simulink model "Prueba_Control_Cuadrupedo_Fisico_Imanes"  (R2025b)
settings: Solver=FixedStepAuto  StartTime=0.0  StopTime=inf  FixedStep=0.01  RelTol=1e-3
values from neighbouring files (symbols this model uses):
  f = figure('Color','w',            'Position',[300 300 900 220],            'Name','Joint Velocity Statistics')    [TABLE.m]
undefined symbols (not defined in the file or in its folder): DiscIntNeverNeededParam
libraries: instrumentlib x2, svdutilitieslib x1, simulink_extras x1
settings Model: PacingRate=0.300000  Creator=ketze  LastModifiedBy=ketze

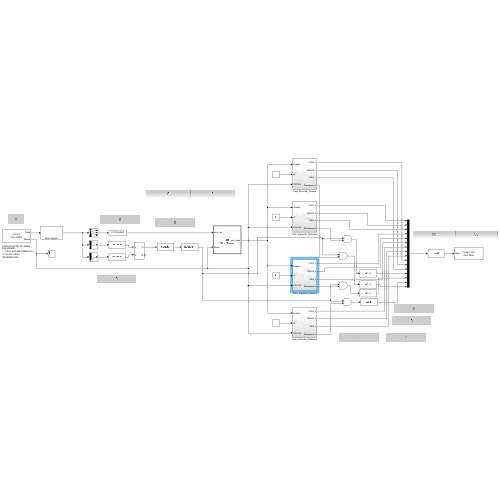
[thumbnail: Simulink's stored preview of the top-level diagram]
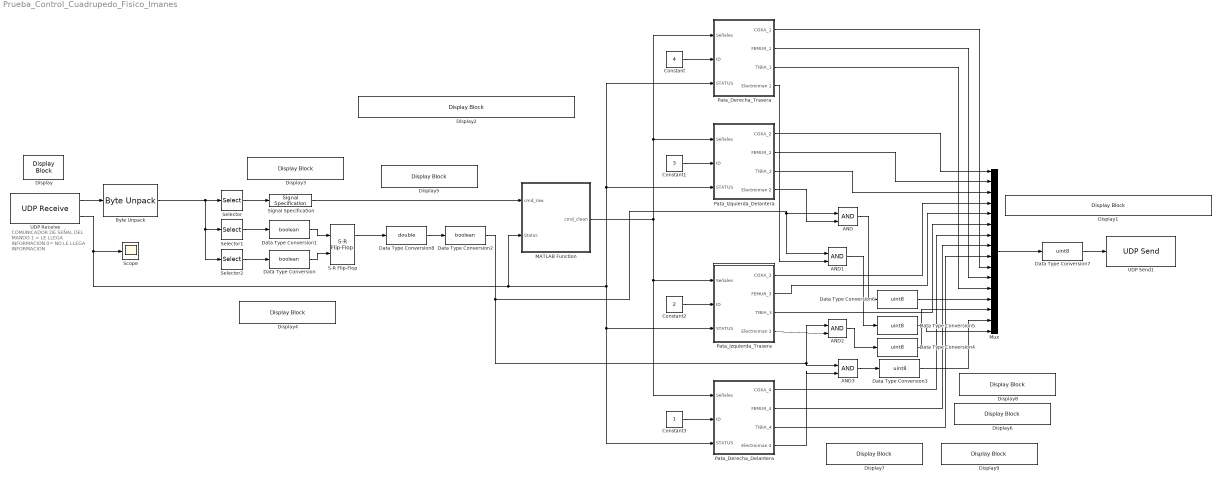
== system Prueba_Control_Cuadrupedo_Fisico_Imanes ==
  note: COMUNICADOR DE SEÑAL DEL MANDO
      | 1 = LE LLEGA INFORMACION
      | 0= NO LE LLEGA INFORMACION
  AND{,1..3} (4 alike) : Logic  IconShape=distinctive  AllPortsSameDT=off  OutDataTypeStr=boolean
  Byte Unpack : svdutilitieslib/Byte Unpack  dimensions={[5]}  datatypes={'double'}  byteAlign=1  blockPlatform=arduinoert
  Constant : Constant  Value=4
  Constant1 : Constant  Value=3
  Constant2 : Constant  Value=2
  Constant3 : Constant
  Data Type Conversion : DataTypeConversion  OutDataTypeStr=boolean  SaturateOnIntegerOverflow=off  RndMeth=Floor
  Data Type Conversion1 : DataTypeConversion  OutDataTypeStr=boolean  SaturateOnIntegerOverflow=off  RndMeth=Floor
  Data Type Conversion2 : DataTypeConversion  OutDataTypeStr=boolean  SaturateOnIntegerOverflow=off  RndMeth=Floor
  Data Type Conversion{3..7} (5 alike) : DataTypeConversion  OutDataTypeStr=uint8  SaturateOnIntegerOverflow=off  RndMeth=Floor
  Data Type Conversion8 : DataTypeConversion  OutDataTypeStr=double  SaturateOnIntegerOverflow=off  RndMeth=Floor
  Display{,1..9} (10 alike) : DisplayBlock  LabelPosition=Hide  Transparency=1  GridColor=[0.502, 0.502, 0.502]
  MATLAB Function : MATLAB Function  TreatAsAtomicUnit=on
  Mux : Mux  Inputs=16
  Pata_Derecha_Delantera : Subsystem
  Pata_Derecha_Trasera : Subsystem
  Pata_Izquierda_Delantera : Subsystem
  Pata_Izquierda_Trasera : Subsystem
  S-R Flip-Flop : simulink_extras/Flip Flops/S-R Flip-Flop  initial_condition=0
  Scope : Scope
  Selector : Selector  InputPortWidth=5  IndexOptions=Index vector (dialog)  Indices=[1 2 3]  OutputSizes=1
  Selector1 : Selector  InputPortWidth=5  IndexOptions=Index vector (dialog)  Indices=[4]  OutputSizes=1
  Selector2 : Selector  InputPortWidth=5  IndexOptions=Index vector (dialog)  Indices=[5]  OutputSizes=1
  Signal Specification : SignalSpecification  Dimensions=3
  UDP Receive : instrumentlib/UDP Receive  LocalAddress=0.0.0.0  LocalPort=25000  EnablePortSharing=off  Host=0.0.0.0  Port=9090  GetLatestData=off  DataSize=40  DataType=uint8  ASCIIFormatting=%f,  Terminator=LF  CustomTerminator=10  ByteOrder=big-endian  EnableBlockingMode=off  Timeout=10  SampleTime=0.02  SimulateUsing=Interpreted execution
  UDP Send1 : instrumentlib/UDP Send  Host=10.46.7.104  Port=5000  LocalAddress=0.0.0.0  LocalPort=-1  EnablePortSharing=off  OutputDatagramPacketSize=512  ByteOrder=big-endian  EnableBlockingMode=on  SimulateUsing=Interpreted execution
  wires:
  Mux/1 -> Data Type Conversion7/1
  Signal Specification/1 -> MATLAB Function/1(cmd_raw)
  UDP Receive/2 -> Scope/1, Pata_Derecha_Trasera/3(STATUS), Pata_Izquierda_Delantera/3(STATUS), Pata_Derecha_Delantera/3(STATUS), Pata_Izquierda_Trasera/3(STATUS), MATLAB Function/2(Status)
  UDP Receive/1 -> Byte Unpack/1
  Constant/1 -> Pata_Derecha_Trasera/2(ID)
  Constant1/1 -> Pata_Izquierda_Delantera/2(ID)
  Constant2/1 -> Pata_Izquierda_Trasera/2(ID)
  Constant3/1 -> Pata_Derecha_Delantera/2(ID)
  MATLAB Function/1(cmd_clean) -> Pata_Derecha_Trasera/1(Señales), Pata_Izquierda_Delantera/1(Señales), Pata_Derecha_Delantera/1(Señales), Pata_Izquierda_Trasera/1(Señales)
  Pata_Izquierda_Delantera/1(COXA_2) -> Mux/1
  Pata_Izquierda_Delantera/2(FEMUR_2) -> Mux/2
  Pata_Izquierda_Delantera/3(TIBIA_2) -> Mux/3
  Pata_Izquierda_Trasera/1(COXA_3) -> Mux/4
  Pata_Izquierda_Trasera/2(FEMUR_3) -> Mux/5
  Pata_Izquierda_Trasera/3(TIBIA_3) -> Mux/6
  Pata_Derecha_Delantera/1(COXA_4) -> Mux/7
  Pata_Derecha_Delantera/2(FEMUR_4) -> Mux/8
  Pata_Derecha_Delantera/3(TIBIA_4) -> Mux/9
  Pata_Derecha_Trasera/1(COXA_1) -> Mux/10
  Pata_Derecha_Trasera/2(FEMUR_1) -> Mux/11
  Pata_Derecha_Trasera/3(TIBIA_1) -> Mux/12
  Selector/1 -> Signal Specification/1
  Selector1/1 -> Data Type Conversion1/1
  Selector2/1 -> Data Type Conversion/1
  S-R Flip-Flop/1 -> Data Type Conversion8/1
  Pata_Izquierda_Delantera/4(Electroiman 2) -> AND/2
  AND/1 -> Data Type Conversion6/1
  Pata_Izquierda_Trasera/4(Electroiman 3) -> AND2/2
  AND2/1 -> Data Type Conversion4/1
  Pata_Derecha_Delantera/4(Electroiman 4) -> AND3/2
  AND3/1 -> Data Type Conversion3/1
  Pata_Derecha_Trasera/4(Electroiman 1) -> AND1/2
  AND1/1 -> Data Type Conversion5/1
  Data Type Conversion1/1 -> S-R Flip-Flop/1
  Data Type Conversion/1 -> S-R Flip-Flop/2
  Data Type Conversion8/1 -> Data Type Conversion2/1
  Data Type Conversion3/1 -> Mux/15
  Data Type Conversion4/1 -> Mux/14
  Data Type Conversion5/1 -> Mux/16
  Data Type Conversion6/1 -> Mux/13
  Data Type Conversion7/1 -> UDP Send1/1
  Byte Unpack/1 -> Selector2/1, Selector1/1, Selector/1
  Data Type Conversion2/1 -> AND3/1, AND2/1, AND1/1, AND/1

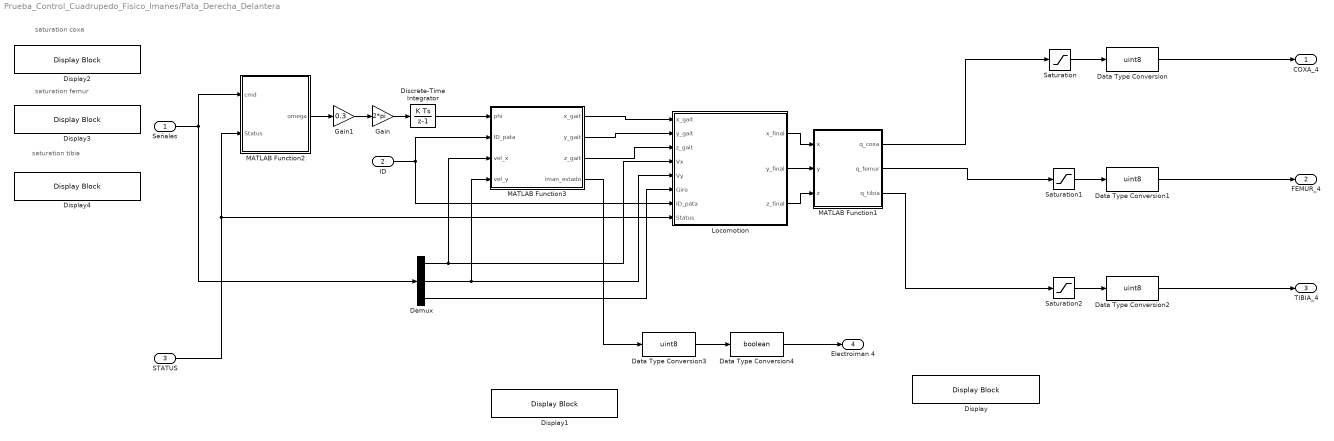
== system Prueba_Control_Cuadrupedo_Fisico_Imanes/Pata_Derecha_Delantera ==
  note: saturation coxa
  note: saturation femur
  note: saturation tibia
  Señales : Inport
  ID : Inport  Port=2
  STATUS : Inport  Port=3
  Data Type Conversion : DataTypeConversion  OutDataTypeStr=uint8  RndMeth=Floor
  Data Type Conversion1 : DataTypeConversion  OutDataTypeStr=uint8  RndMeth=Floor
  Data Type Conversion2 : DataTypeConversion  OutDataTypeStr=uint8  RndMeth=Floor
  Data Type Conversion3 : DataTypeConversion  OutDataTypeStr=uint8  SaturateOnIntegerOverflow=off  RndMeth=Floor
  Data Type Conversion4 : DataTypeConversion  OutDataTypeStr=boolean  SaturateOnIntegerOverflow=off  RndMeth=Floor
  Demux : Demux  Outputs=3
  Discrete-Time Integrator : DiscreteIntegrator  SampleTime=0.01  ICPrevOutput=DiscIntNeverNeededParam  ICPrevScaledInput=DiscIntNeverNeededParam
  Display{,1..4} (5 alike) : DisplayBlock  LabelPosition=Hide  Transparency=1  GridColor=[0.502, 0.502, 0.502]
  Gain : Gain  Gain=2*pi
  Gain1 : Gain  Gain=0.3
  Locomotion : MATLAB Function  TreatAsAtomicUnit=on
  MATLAB Function1 : MATLAB Function  TreatAsAtomicUnit=on
  MATLAB Function2 : MATLAB Function  TreatAsAtomicUnit=on
  MATLAB Function3 : MATLAB Function  TreatAsAtomicUnit=on
  Saturation : Saturate  UpperLimit=180  LowerLimit=0
  Saturation1 : Saturate  UpperLimit=180  LowerLimit=0
  Saturation2 : Saturate  UpperLimit=180  LowerLimit=0
  COXA_4 : Outport
  FEMUR_4 : Outport  Port=2
  TIBIA_4 : Outport  Port=3
  Electroiman 4 : Outport  Port=4
  wires:
  MATLAB Function1/1(q_coxa) -> Saturation/1
  MATLAB Function1/2(q_femur) -> Saturation1/1
  MATLAB Function1/3(q_tibia) -> Saturation2/1
  Saturation/1 -> Data Type Conversion/1
  Saturation1/1 -> Data Type Conversion1/1
  Saturation2/1 -> Data Type Conversion2/1
  Locomotion/1(x_final) -> MATLAB Function1/1(x)
  Señales/1 -> Demux/1, MATLAB Function2/1(cmd)
  Gain/1 -> Discrete-Time Integrator/1
  STATUS/1 -> Locomotion/8(Status), MATLAB Function2/2(Status)
  Demux/1 -> Locomotion/4(Vx), MATLAB Function3/3(vel_x)
  ID/1 -> Locomotion/7(ID_pata), MATLAB Function3/2(ID_pata)
  MATLAB Function2/1(omega) -> Gain1/1
  Demux/2 -> MATLAB Function3/4(vel_y), Locomotion/5(Vy)
  MATLAB Function3/3(z_gait) -> Locomotion/3(z_gait)
  MATLAB Function3/2(y_gait) -> Locomotion/2(y_gait)
  MATLAB Function3/1(x_gait) -> Locomotion/1(x_gait)
  Locomotion/2(y_final) -> MATLAB Function1/2(y)
  Demux/3 -> Locomotion/6(Giro)
  Locomotion/3(z_final) -> MATLAB Function1/3(z)
  MATLAB Function3/4(iman_estado) -> Data Type Conversion3/1
  Data Type Conversion3/1 -> Data Type Conversion4/1
  Discrete-Time Integrator/1 -> MATLAB Function3/1(phi)
  Gain1/1 -> Gain/1
  Data Type Conversion2/1 -> TIBIA_4/1
  Data Type Conversion1/1 -> FEMUR_4/1
  Data Type Conversion/1 -> COXA_4/1
  Data Type Conversion4/1 -> Electroiman 4/1

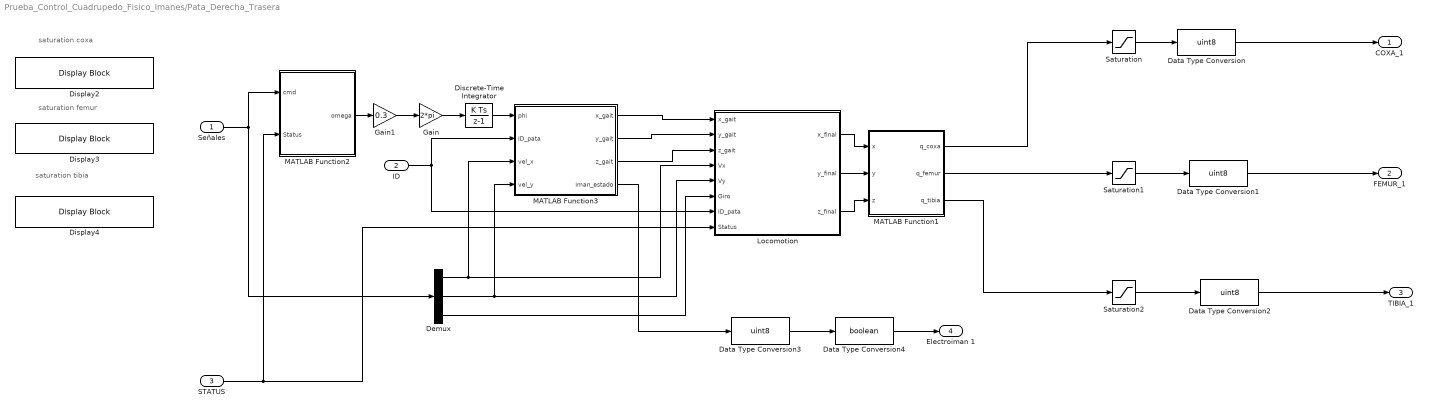
== system Prueba_Control_Cuadrupedo_Fisico_Imanes/Pata_Derecha_Trasera ==
  note: saturation coxa
  note: saturation femur
  note: saturation tibia
  Señales : Inport
  ID : Inport  Port=2
  STATUS : Inport  Port=3
  Data Type Conversion : DataTypeConversion  OutDataTypeStr=uint8  RndMeth=Floor
  Data Type Conversion1 : DataTypeConversion  OutDataTypeStr=uint8  RndMeth=Floor
  Data Type Conversion2 : DataTypeConversion  OutDataTypeStr=uint8  RndMeth=Floor
  Data Type Conversion3 : DataTypeConversion  OutDataTypeStr=uint8  SaturateOnIntegerOverflow=off  RndMeth=Floor
  Data Type Conversion4 : DataTypeConversion  OutDataTypeStr=boolean  SaturateOnIntegerOverflow=off  RndMeth=Floor
  Demux : Demux  Outputs=3
  Discrete-Time Integrator : DiscreteIntegrator  SampleTime=0.01  ICPrevOutput=DiscIntNeverNeededParam  ICPrevScaledInput=DiscIntNeverNeededParam
  Display2 : DisplayBlock  LabelPosition=Hide  Transparency=1  GridColor=[0.502, 0.502, 0.502]
  Display3 : DisplayBlock  LabelPosition=Hide  Transparency=1  GridColor=[0.502, 0.502, 0.502]
  Display4 : DisplayBlock  LabelPosition=Hide  Transparency=1  GridColor=[0.502, 0.502, 0.502]
  Gain : Gain  Gain=2*pi
  Gain1 : Gain  Gain=0.3
  Locomotion : MATLAB Function  TreatAsAtomicUnit=on
  MATLAB Function1 : MATLAB Function  TreatAsAtomicUnit=on
  MATLAB Function2 : MATLAB Function  TreatAsAtomicUnit=on
  MATLAB Function3 : MATLAB Function  TreatAsAtomicUnit=on
  Saturation : Saturate  UpperLimit=180  LowerLimit=0
  Saturation1 : Saturate  UpperLimit=180  LowerLimit=0
  Saturation2 : Saturate  UpperLimit=180  LowerLimit=0
  COXA_1 : Outport
  FEMUR_1 : Outport  Port=2
  TIBIA_1 : Outport  Port=3
  Electroiman 1 : Outport  Port=4
  wires:
  MATLAB Function1/1(q_coxa) -> Saturation/1
  MATLAB Function1/2(q_femur) -> Saturation1/1
  MATLAB Function1/3(q_tibia) -> Saturation2/1
  Saturation/1 -> Data Type Conversion/1
  Saturation1/1 -> Data Type Conversion1/1
  Saturation2/1 -> Data Type Conversion2/1
  Demux/3 -> Locomotion/6(Giro)
  Locomotion/3(z_final) -> MATLAB Function1/3(z)
  Demux/1 -> Locomotion/4(Vx), MATLAB Function3/3(vel_x)
  Locomotion/2(y_final) -> MATLAB Function1/2(y)
  MATLAB Function2/1(omega) -> Gain1/1
  MATLAB Function3/3(z_gait) -> Locomotion/3(z_gait)
  Demux/2 -> MATLAB Function3/4(vel_y), Locomotion/5(Vy)
  MATLAB Function3/2(y_gait) -> Locomotion/2(y_gait)
  ID/1 -> Locomotion/7(ID_pata), MATLAB Function3/2(ID_pata)
  Señales/1 -> Demux/1, MATLAB Function2/1(cmd)
  Locomotion/1(x_final) -> MATLAB Function1/1(x)
  Gain/1 -> Discrete-Time Integrator/1
  MATLAB Function3/1(x_gait) -> Locomotion/1(x_gait)
  STATUS/1 -> Locomotion/8(Status), MATLAB Function2/2(Status)
  MATLAB Function3/4(iman_estado) -> Data Type Conversion3/1
  Data Type Conversion3/1 -> Data Type Conversion4/1
  Discrete-Time Integrator/1 -> MATLAB Function3/1(phi)
  Gain1/1 -> Gain/1
  Data Type Conversion/1 -> COXA_1/1
  Data Type Conversion1/1 -> FEMUR_1/1
  Data Type Conversion2/1 -> TIBIA_1/1
  Data Type Conversion4/1 -> Electroiman 1/1

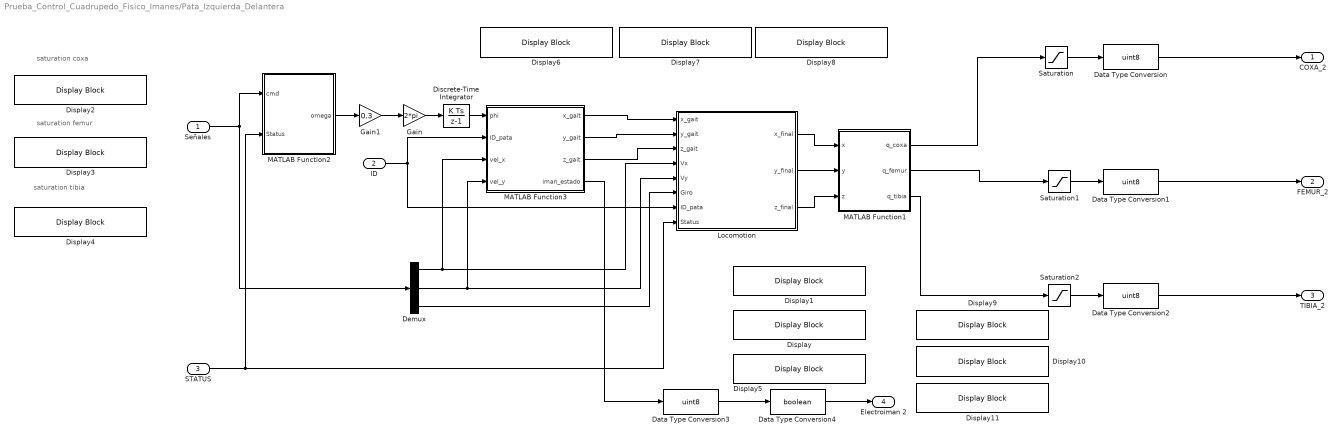
== system Prueba_Control_Cuadrupedo_Fisico_Imanes/Pata_Izquierda_Delantera ==
  note: saturation coxa
  note: saturation femur
  note: saturation tibia
  Señales : Inport
  ID : Inport  Port=2
  STATUS : Inport  Port=3
  Data Type Conversion : DataTypeConversion  OutDataTypeStr=uint8  RndMeth=Floor
  Data Type Conversion1 : DataTypeConversion  OutDataTypeStr=uint8  RndMeth=Floor
  Data Type Conversion2 : DataTypeConversion  OutDataTypeStr=uint8  RndMeth=Floor
  Data Type Conversion3 : DataTypeConversion  OutDataTypeStr=uint8  SaturateOnIntegerOverflow=off  RndMeth=Floor
  Data Type Conversion4 : DataTypeConversion  OutDataTypeStr=boolean  SaturateOnIntegerOverflow=off  RndMeth=Floor
  Demux : Demux  Outputs=3
  Discrete-Time Integrator : DiscreteIntegrator  SampleTime=0.01  ICPrevOutput=DiscIntNeverNeededParam  ICPrevScaledInput=DiscIntNeverNeededParam
  Display{,1..11} (12 alike) : DisplayBlock  LabelPosition=Hide  Transparency=1  GridColor=[0.502, 0.502, 0.502]
  Gain : Gain  Gain=2*pi
  Gain1 : Gain  Gain=0.3
  Locomotion : MATLAB Function  TreatAsAtomicUnit=on
  MATLAB Function1 : MATLAB Function  TreatAsAtomicUnit=on
  MATLAB Function2 : MATLAB Function  TreatAsAtomicUnit=on
  MATLAB Function3 : MATLAB Function  TreatAsAtomicUnit=on
  Saturation : Saturate  UpperLimit=180  LowerLimit=0
  Saturation1 : Saturate  UpperLimit=180  LowerLimit=0
  Saturation2 : Saturate  UpperLimit=180  LowerLimit=0
  COXA_2 : Outport
  FEMUR_2 : Outport  Port=2
  TIBIA_2 : Outport  Port=3
  Electroiman 2 : Outport  Port=4
  wires:
  MATLAB Function1/1(q_coxa) -> Saturation/1
  MATLAB Function1/2(q_femur) -> Saturation1/1
  MATLAB Function1/3(q_tibia) -> Saturation2/1
  Saturation/1 -> Data Type Conversion/1
  Saturation1/1 -> Data Type Conversion1/1
  Saturation2/1 -> Data Type Conversion2/1
  Locomotion/1(x_final) -> MATLAB Function1/1(x)
  Señales/1 -> Demux/1, MATLAB Function2/1(cmd)
  Gain/1 -> Discrete-Time Integrator/1
  STATUS/1 -> Locomotion/8(Status), MATLAB Function2/2(Status)
  Demux/1 -> Locomotion/4(Vx), MATLAB Function3/3(vel_x)
  ID/1 -> Locomotion/7(ID_pata), MATLAB Function3/2(ID_pata)
  MATLAB Function2/1(omega) -> Gain1/1
  Demux/2 -> MATLAB Function3/4(vel_y), Locomotion/5(Vy)
  MATLAB Function3/3(z_gait) -> Locomotion/3(z_gait)
  MATLAB Function3/2(y_gait) -> Locomotion/2(y_gait)
  MATLAB Function3/1(x_gait) -> Locomotion/1(x_gait)
  Locomotion/2(y_final) -> MATLAB Function1/2(y)
  Demux/3 -> Locomotion/6(Giro)
  Locomotion/3(z_final) -> MATLAB Function1/3(z)
  MATLAB Function3/4(iman_estado) -> Data Type Conversion3/1
  Data Type Conversion3/1 -> Data Type Conversion4/1
  Discrete-Time Integrator/1 -> MATLAB Function3/1(phi)
  Gain1/1 -> Gain/1
  Data Type Conversion/1 -> COXA_2/1
  Data Type Conversion1/1 -> FEMUR_2/1
  Data Type Conversion2/1 -> TIBIA_2/1
  Data Type Conversion4/1 -> Electroiman 2/1

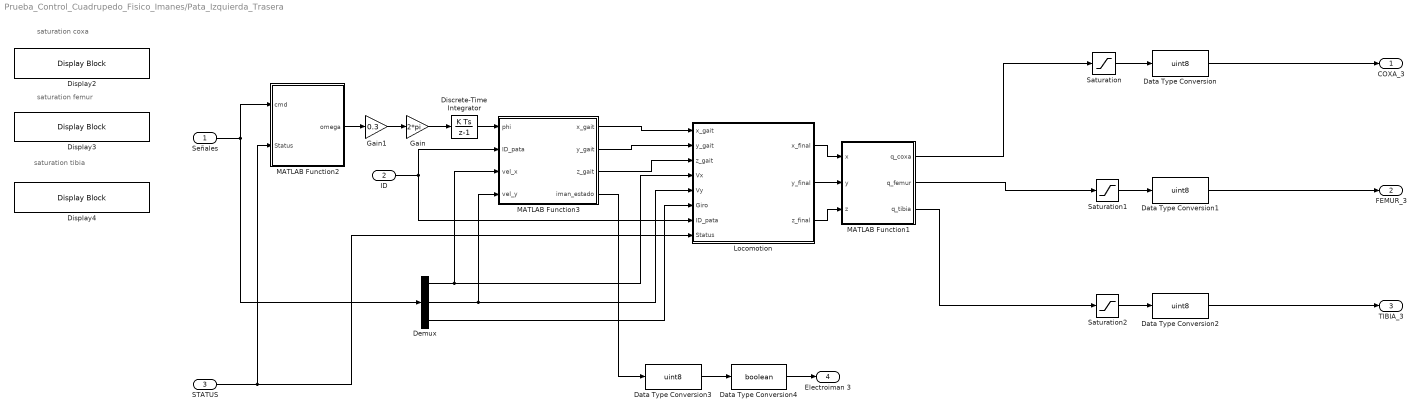
== system Prueba_Control_Cuadrupedo_Fisico_Imanes/Pata_Izquierda_Trasera ==
  note: saturation coxa
  note: saturation femur
  note: saturation tibia
  Señales : Inport
  ID : Inport  Port=2
  STATUS : Inport  Port=3
  Data Type Conversion : DataTypeConversion  OutDataTypeStr=uint8  RndMeth=Floor
  Data Type Conversion1 : DataTypeConversion  OutDataTypeStr=uint8  RndMeth=Floor
  Data Type Conversion2 : DataTypeConversion  OutDataTypeStr=uint8  RndMeth=Floor
  Data Type Conversion3 : DataTypeConversion  OutDataTypeStr=uint8  SaturateOnIntegerOverflow=off  RndMeth=Floor
  Data Type Conversion4 : DataTypeConversion  OutDataTypeStr=boolean  SaturateOnIntegerOverflow=off  RndMeth=Floor
  Demux : Demux  Outputs=3
  Discrete-Time Integrator : DiscreteIntegrator  SampleTime=0.01  ICPrevOutput=DiscIntNeverNeededParam  ICPrevScaledInput=DiscIntNeverNeededParam
  Display2 : DisplayBlock  LabelPosition=Hide  Transparency=1  GridColor=[0.502, 0.502, 0.502]
  Display3 : DisplayBlock  LabelPosition=Hide  Transparency=1  GridColor=[0.502, 0.502, 0.502]
  Display4 : DisplayBlock  LabelPosition=Hide  Transparency=1  GridColor=[0.502, 0.502, 0.502]
  Gain : Gain  Gain=2*pi
  Gain1 : Gain  Gain=0.3
  Locomotion : MATLAB Function  TreatAsAtomicUnit=on
  MATLAB Function1 : MATLAB Function  TreatAsAtomicUnit=on
  MATLAB Function2 : MATLAB Function  TreatAsAtomicUnit=on
  MATLAB Function3 : MATLAB Function  TreatAsAtomicUnit=on
  Saturation : Saturate  UpperLimit=180  LowerLimit=0
  Saturation1 : Saturate  UpperLimit=180  LowerLimit=0
  Saturation2 : Saturate  UpperLimit=180  LowerLimit=0
  COXA_3 : Outport
  FEMUR_3 : Outport  Port=2
  TIBIA_3 : Outport  Port=3
  Electroiman 3 : Outport  Port=4
  wires:
  MATLAB Function1/1(q_coxa) -> Saturation/1
  MATLAB Function1/2(q_femur) -> Saturation1/1
  MATLAB Function1/3(q_tibia) -> Saturation2/1
  Saturation/1 -> Data Type Conversion/1
  Saturation1/1 -> Data Type Conversion1/1
  Saturation2/1 -> Data Type Conversion2/1
  Locomotion/1(x_final) -> MATLAB Function1/1(x)
  Señales/1 -> Demux/1, MATLAB Function2/1(cmd)
  Gain/1 -> Discrete-Time Integrator/1
  STATUS/1 -> Locomotion/8(Status), MATLAB Function2/2(Status)
  Demux/1 -> Locomotion/4(Vx), MATLAB Function3/3(vel_x)
  ID/1 -> Locomotion/7(ID_pata), MATLAB Function3/2(ID_pata)
  MATLAB Function2/1(omega) -> Gain1/1
  Demux/2 -> MATLAB Function3/4(vel_y), Locomotion/5(Vy)
  MATLAB Function3/3(z_gait) -> Locomotion/3(z_gait)
  MATLAB Function3/2(y_gait) -> Locomotion/2(y_gait)
  MATLAB Function3/1(x_gait) -> Locomotion/1(x_gait)
  Locomotion/2(y_final) -> MATLAB Function1/2(y)
  Demux/3 -> Locomotion/6(Giro)
  Locomotion/3(z_final) -> MATLAB Function1/3(z)
  MATLAB Function3/4(iman_estado) -> Data Type Conversion3/1
  Data Type Conversion3/1 -> Data Type Conversion4/1
  Discrete-Time Integrator/1 -> MATLAB Function3/1(phi)
  Gain1/1 -> Gain/1
  Data Type Conversion2/1 -> TIBIA_3/1
  Data Type Conversion1/1 -> FEMUR_3/1
  Data Type Conversion/1 -> COXA_3/1
  Data Type Conversion4/1 -> Electroiman 3/1

== matlab function Prueba_Control_Cuadrupedo_Fisico_Imanes/Pata_Derecha_Delantera/Locomotion ==
  data: x_gait input; x_final output; y_gait input; z_gait input; Vx input; Vy input; Giro input; ID_pata input; y_final output; z_final output; Status input
function [x_final, y_final, z_final] = fcn(x_gait, y_gait, z_gait, Vx, Vy, Giro, ID_pata, Status)
    
    % --- 1. CONVERSIÓN SEGURA (CORTAFUEGOS) ---
    Vx_d = double(Vx(1));
    Vy_d = double(Vy(1));
    Giro_d = double(Giro(1));
    
    % --- 2. MEMORIA DEL MANDO ---
    persistent Vx_last Vy_last Giro_last
    if isempty(Vx_last)
        Vx_last = 0; Vy_last = 0; Giro_last = 0; 
    end
    
    if logical(Status) == true
        Vx_last = Vx_d;
        Vy_last = Vy_d;
        Giro_last = Giro_d;
    end
    
    % --- 3. FILTRO SUAVIZADOR (ANTI-TEMBLORES) ---
    persistent Vx_f Vy_f Giro_f
    if isempty(Vx_f)
        Vx_f = 0; Vy_f = 0; Giro_f = 0;
    end
    
    % Alpha en 0.15 actúa como amortiguador. Ya no saltará violentamente.
    alpha = 0.15; 
    Vx_f = (1-alpha)*Vx_f + alpha*Vx_last;
    Vy_f = (1-alpha)*Vy_f + alpha*Vy_last;
    Giro_f = (1-alpha)*Giro_f + alpha*Giro_last;
    
    % --- 4. CINEMÁTICA DEL CUERPO Y SALIDA ---
    % Como el gait_generator ya calcula la zancada con vel_x y vel_y,
    % Locomotion solo debe aplicar pequeñas correcciones de postura 
    % o pasar la trayectoria limpia para no deformar el paso.
    
    % Por ahora, pasamos la trayectoria limpia del generador de marcha.
    % Si en el futuro quieres que el cuerpo se incline (body kinematics),
    % se sumaría aquí.
    
    x_final = x_gait;
    y_final = y_gait;
    z_final = z_gait;
end

== matlab function Prueba_Control_Cuadrupedo_Fisico_Imanes/Pata_Derecha_Trasera/MATLAB Function2 ==
  data: cmd input; omega output; Status input
function omega = gait_speed(cmd, Status)
    
    % --- 1. MEMORIA CONTRA EL PARPADEO ---
    persistent cmd_last
    if isempty(cmd_last)
        cmd_last = zeros(3, 1, 'single'); 
    end
    
    if logical(Status) == true
        cmd_last = single(cmd(:)); 
    end
    
    % --- 2. LEER DE LA MEMORIA Y CONVERTIR ---
    % ¡Aquí está el truco! Pasamos al formato 'double' de una vez
    % para que todas las matemáticas fluyan sin errores.
    Vx = double(cmd_last(1));
    Vy = double(cmd_last(2));
    Wz = double(cmd_last(3));
    
    % --- 3. CÁLCULO DE VELOCIDAD ---
    % Ahora 'vel' nace siendo double
    vel = sqrt(Vx^2 + Vy^2 + Wz^2);
    
    % zona muerta
    if vel < 0.1
        vel = 0; % Como 'vel' y '0' son double, ya no hay choque
    end
    
    % frecuencia base del gait
    freq_max = 1.5; 
    omega = vel * freq_max;

== matlab function Prueba_Control_Cuadrupedo_Fisico_Imanes/Pata_Derecha_Trasera/MATLAB Function3 ==
  data: phi input; x_gait output; ID_pata input; y_gait output; z_gait output; vel_x input; vel_y input; iman_estado output
function [x_gait, y_gait, z_gait, iman_estado] = gait_generator(phi, ID_pata, vel_x, vel_y)
% --- 1. POSTURA BASE Y LÍMITES ---
BASE_X = 150;
NOMINAL_Z = -130;
% --- CONFIGURACIÓN DE ALTURA DE PASO UNIFICADA ---
LIFT_Z = -70;
Y_ATRAS = -40;
Y_ADELANTE = 40;
% --- 2. NORMALIZAR EL CICLO Y ORDEN DE MARCHA ---
t_norm = mod(phi, 2*pi) / (2*pi);
switch ID_pata
case 1 % Pata Derecha Delantera
offset = 0.0;
case 2 % Pata Izquierda Trasera
offset = 0.25;
case 3 % Pata Izquierda Delantera
offset = 0.50;
case 4 % Pata Derecha Trasera
offset = 0.75;
otherwise
offset = 0.0;
end
p_local = mod(t_norm - offset, 1.0);
% --- 3. TRAYECTORIA EN 4 FASES (MOVIMIENTO ACTIVO) ---
x_gait = BASE_X;
% FASE 1: DESPEGUE Y VUELO
if p_local < 0.20
s = p_local / 0.20;
s_smooth = 0.5 * (1 - cos(s * pi));
y_gait = Y_ATRAS + (Y_ADELANTE - Y_ATRAS) * s_smooth;
z_gait = NOMINAL_Z + (NOMINAL_Z - LIFT_Z) * -sin(s * pi);
iman_estado_calculado = 0;
% FASE 2: ATERRIZAJE Y ANCLAJE
elseif p_local < 0.25
y_gait = Y_ADELANTE;
z_gait = NOMINAL_Z;
iman_estado_calculado = 1;
% FASE 3: EMPUJE / STANCE
elseif p_local < 0.95
s = (p_local - 0.25) / 0.70;
y_gait = Y_ADELANTE - (Y_ADELANTE - Y_ATRAS) * s;
z_gait = NOMINAL_Z + 10; % Corrección geométrica vertical fija para esta pata
iman_estado_calculado = 1;
% FASE 4: LIBERACIÓN DEL IMÁN
else
y_gait = Y_ATRAS;
z_gait = NOMINAL_Z + 10; % Corrección geométrica vertical fija para esta pata
iman_estado_calculado = 0;
end
% --- 4. CORTAFUEGOS INTELIGENTE: MODO STANDBY TOTAL ---
if abs(vel_x) < 0.1 && abs(vel_y) < 0.1
    x_gait = BASE_X;
    y_gait = 0;
    z_gait = NOMINAL_Z + 10; % Mantiene su altura corregida en reposo
    
    % SOLUCCIÓN DEFINITIVA: Cuando el robot se detiene por completo,
    % obligamos a que el imán se encienda (1) para garantizar que las 4 patas
    % queden totalmente ancladas al suelo en modo estacionario.
    iman_estado = 1; 
    return;
else
    % En movimiento dinámico, sigue la secuencia matemática de las fases
    iman_estado = iman_estado_calculado;
end
end

== matlab function Prueba_Control_Cuadrupedo_Fisico_Imanes/Pata_Izquierda_Trasera/MATLAB Function1 ==
  data: x input; q_coxa output; y input; z input; q_femur output; q_tibia output
function [q_coxa, q_femur, q_tibia] = InverseKinematics(x, y, z)
    % --- 1. CONFIGURACIÓN DEL ROBOT ---
    L1 = 56.84;  % Coxa
    L2 = 80.37;  % Fémur
    L3 = 187.3;  % Tibia 
    
    % --- 2. AJUSTES MANUALES ---
    % Vamos a restar unos 80 grados de golpe para bajar la tibia
    OFFSET_TIBIA = -130;  % (Antes estaba en -40)
    
    % Y por si acaso, bajemos un poco el fémur también
    OFFSET_FEMUR = 30;    % (Antes estaba en 60)
    
    % (Si la tibia izquierda necesita un toque extra de calibración, muévelo aquí)
    AJUSTE_FINO_FEMUR_IZQ = -22;
    AJUSTE_FINO_TIBIA_IZQ = -5; 
    
    % --- 3. CÁLCULOS ---
    q_coxa_rad = -atan2(y, x); 
    distancia_xy = sqrt(x^2 + y^2);
    
    R = distancia_xy - L1;
    D = sqrt(R^2 + z^2);
    
    % --- 4. PROTECCIÓN MATEMÁTICA ---
    if D > (L2 + L3)
        D = L2 + L3; 
    end
    D = max(D, abs(L2 - L3) + 1);
    
    cos_alfa = (L2^2 + D^2 - L3^2) / (2 * L2 * D);
    cos_beta = (L2^2 + L3^2 - D^2) / (2 * L2 * L3);
    
    alfa = acos(max(min(cos_alfa, 1), -1));
    beta = acos(max(min(cos_beta, 1), -1));
    elevacion = atan2(z, R); 
    
    % --- 5. CÁLCULO DE ÁNGULOS EN RADIANES ---
    q_femur_rad = -(alfa + elevacion); 
    q_tibia_rad = (pi - beta);         
    
    % --- 6. SALIDA FINAL INVERTIDA (CORREGIDA) ---
   femur_derecho = rad2deg(q_femur_rad) + OFFSET_FEMUR + 90;
    tibia_derecha = rad2deg(q_tibia_rad) + OFFSET_TIBIA + 90;
    
    q_coxa  = rad2deg(q_coxa_rad) + 90; 

    % Le sumamos el ajuste fino directamente aquí afuera del espejo:
    q_femur = (180 - femur_derecho) + AJUSTE_FINO_FEMUR_IZQ; 
    q_tibia = (180 - tibia_derecha) + AJUSTE_FINO_TIBIA_IZQ;
    
    % --- 7. CORTAFUEGOS DE SEGURIDAD (ANTI-COLAPSO) ---
    % Esto asegura que jamás se envíe un número que rompa el uint8
    if q_tibia < 5
        q_tibia = 5;
    elseif q_tibia > 175
        q_tibia = 175;
    end
    
    if q_femur < 5
        q_femur = 5;
    elseif q_femur > 175
        q_femur = 175;
    end
end

== matlab function Prueba_Control_Cuadrupedo_Fisico_Imanes/Pata_Izquierda_Trasera/MATLAB Function2 ==
  data: cmd input; omega output; Status input
function omega = gait_speed(cmd, Status)
    
    % --- 1. MEMORIA CONTRA EL PARPADEO ---
    persistent cmd_last
    if isempty(cmd_last)
        cmd_last = zeros(3, 1, 'single'); 
    end
    
    if logical(Status) == true
        cmd_last = single(cmd(:)); 
    end
    
    % --- 2. LEER DE LA MEMORIA Y CONVERTIR ---
    % ¡Aquí está el truco! Pasamos al formato 'double' de una vez
    % para que todas las matemáticas fluyan sin errores.
    Vx = double(cmd_last(1));
    Vy = double(cmd_last(2));
    Wz = double(cmd_last(3));
    
    % --- 3. CÁLCULO DE VELOCIDAD ---
    % Ahora 'vel' nace siendo double
    vel = sqrt(Vx^2 + Vy^2 + Wz^2);
    
    % zona muerta
    if vel < 0.1
        vel = 0; % Como 'vel' y '0' son double, ya no hay choque
    end
    
    % frecuencia base del gait
    freq_max = 1.5; 
    omega = vel * freq_max;

== matlab function Prueba_Control_Cuadrupedo_Fisico_Imanes/Pata_Derecha_Trasera/Locomotion ==
  data: x_gait input; x_final output; y_gait input; z_gait input; Vx input; Vy input; Giro input; ID_pata input; y_final output; z_final output; Status input
function [x_final, y_final, z_final] = fcn(x_gait, y_gait, z_gait, Vx, Vy, Giro, ID_pata, Status)
    
    % --- 1. CONVERSIÓN SEGURA (CORTAFUEGOS) ---
    Vx_d = double(Vx(1));
    Vy_d = double(Vy(1));
    Giro_d = double(Giro(1));
    
    % --- 2. MEMORIA DEL MANDO ---
    persistent Vx_last Vy_last Giro_last
    if isempty(Vx_last)
        Vx_last = 0; Vy_last = 0; Giro_last = 0; 
    end
    
    if logical(Status) == true
        Vx_last = Vx_d;
        Vy_last = Vy_d;
        Giro_last = Giro_d;
    end
    
    % --- 3. FILTRO SUAVIZADOR (ANTI-TEMBLORES) ---
    persistent Vx_f Vy_f Giro_f
    if isempty(Vx_f)
        Vx_f = 0; Vy_f = 0; Giro_f = 0;
    end
    
    % Alpha en 0.15 actúa como amortiguador. Ya no saltará violentamente.
    alpha = 0.15; 
    Vx_f = (1-alpha)*Vx_f + alpha*Vx_last;
    Vy_f = (1-alpha)*Vy_f + alpha*Vy_last;
    Giro_f = (1-alpha)*Giro_f + alpha*Giro_last;
    
    % --- 4. CINEMÁTICA DEL CUERPO Y SALIDA ---
    % Como el gait_generator ya calcula la zancada con vel_x y vel_y,
    % Locomotion solo debe aplicar pequeñas correcciones de postura 
    % o pasar la trayectoria limpia para no deformar el paso.
    
    % Por ahora, pasamos la trayectoria limpia del generador de marcha.
    % Si en el futuro quieres que el cuerpo se incline (body kinematics),
    % se sumaría aquí.
    
    x_final = x_gait;
    y_final = y_gait;
    z_final = z_gait;
end

== matlab function Prueba_Control_Cuadrupedo_Fisico_Imanes/Pata_Izquierda_Trasera/MATLAB Function3 ==
  data: phi input; x_gait output; ID_pata input; y_gait output; z_gait output; vel_x input; vel_y input; iman_estado output
function [x_gait, y_gait, z_gait, iman_estado] = gait_generator(phi, ID_pata, vel_x, vel_y)
% --- 1. POSTURA BASE Y LÍMITES ---
BASE_X = 150;
NOMINAL_Z = -130;
% --- CONFIGURACIÓN DE ALTURA DE PASO UNIFICADA ---
LIFT_Z = -70;
Y_ATRAS = -40;
Y_ADELANTE = 40;
% --- 2. NORMALIZAR EL CICLO Y ORDEN DE MARCHA ---
t_norm = mod(phi, 2*pi) / (2*pi);
switch ID_pata
case 1 % Pata Derecha Delantera
offset = 0.0;
case 2 % Pata Izquierda Trasera
offset = 0.25;
case 3 % Pata Izquierda Delantera
offset = 0.50;
case 4 % Pata Derecha Trasera
offset = 0.75;
otherwise
offset = 0.0;
end
p_local = mod(t_norm - offset, 1.0);
% --- 3. TRAYECTORIA EN 4 FASES (MOVIMIENTO ACTIVO) ---
x_gait = BASE_X;
% FASE 1: DESPEGUE Y VUELO
if p_local < 0.20
s = p_local / 0.20;
s_smooth = 0.5 * (1 - cos(s * pi));
y_gait = Y_ATRAS + (Y_ADELANTE - Y_ATRAS) * s_smooth;
z_gait = NOMINAL_Z + (NOMINAL_Z - LIFT_Z) * -sin(s * pi);
iman_estado_calculado = 0;
% FASE 2: ATERRIZAJE Y ANCLAJE
elseif p_local < 0.25
y_gait = Y_ADELANTE;
z_gait = NOMINAL_Z;
iman_estado_calculado = 1;
% FASE 3: EMPUJE / STANCE
elseif p_local < 0.95
s = (p_local - 0.25) / 0.70;
y_gait = Y_ADELANTE - (Y_ADELANTE - Y_ATRAS) * s;
z_gait = NOMINAL_Z + 10; % Corrección geométrica vertical fija para esta pata
iman_estado_calculado = 1;
% FASE 4: LIBERACIÓN DEL IMÁN
else
y_gait = Y_ATRAS;
z_gait = NOMINAL_Z + 10; % Corrección geométrica vertical fija para esta pata
iman_estado_calculado = 0;
end
% --- 4. CORTAFUEGOS INTELIGENTE: MODO STANDBY TOTAL ---
if abs(vel_x) < 0.1 && abs(vel_y) < 0.1
    x_gait = BASE_X;
    y_gait = 0;
    z_gait = NOMINAL_Z + 10; % Mantiene su altura corregida en reposo
    
    % SOLUCCIÓN DEFINITIVA: Cuando el robot se detiene por completo,
    % obligamos a que el imán se encienda (1) para garantizar que las 4 patas
    % queden totalmente ancladas al suelo en modo estacionario.
    iman_estado = 1; 
    return;
else
    % En movimiento dinámico, sigue la secuencia matemática de las fases
    iman_estado = iman_estado_calculado;
end
end

== matlab function Prueba_Control_Cuadrupedo_Fisico_Imanes/Pata_Derecha_Delantera/MATLAB Function1 ==
  data: x input; q_coxa output; y input; z input; q_femur output; q_tibia output
function [q_coxa, q_femur, q_tibia] = InverseKinematics(x, y, z)
    % --- 1. CONFIGURACIÓN DEL ROBOT ---
    L1 = 56.84;  % Coxa
    L2 = 80.37;  % Fémur
    L3 = 187.3;  % Tibia 
    
    % --- 2. AJUSTES MANUALES ---
    % Vamos a restar unos 80 grados de golpe para bajar la tibia
    OFFSET_TIBIA = -110;  % (Antes estaba en -40)
    
    % Y por si acaso, bajemos un poco el fémur también
    OFFSET_FEMUR = 60;    % (Antes estaba en 60)
    
    % Mantenemos el ajuste del fémur que ya te funcionó perfecto:
    AJUSTE_FINO_FEMUR_DER = -15; 
    
    % (Agregamos esta nueva variable para bajar la tibia y que toque el piso)
    % Probamos con 20 grados positivos para que la tibia gire hacia abajo
    AJUSTE_FINO_TIBIA_DER = -15; 
    
    % --- 3. CÁLCULOS ---
    q_coxa_rad = -atan2(y, x); 
    distancia_xy = sqrt(x^2 + y^2);
    
    R = distancia_xy - L1;
    D = sqrt(R^2 + z^2);
    
    % --- 4. PROTECCIÓN MATEMÁTICA ---
    if D > (L2 + L3)
        D = L2 + L3; 
    end
    D = max(D, abs(L2 - L3) + 1);
    
    cos_alfa = (L2^2 + D^2 - L3^2) / (2 * L2 * D);
    cos_beta = (L2^2 + L3^2 - D^2) / (2 * L2 * L3);
    
    alfa = acos(max(min(cos_alfa, 1), -1));
    beta = acos(max(min(cos_beta, 1), -1));
    elevacion = atan2(z, R); 
    
    % --- 5. CÁLCULO DE ÁNGULOS EN RADIANES ---
    q_femur_rad = -(alfa + elevacion); 
    q_tibia_rad = (pi - beta);         
    
    % --- 6. SALIDA FINAL NORMAL (LADO DERECHO PCA 0x41) ---
    q_coxa  = rad2deg(q_coxa_rad) + 90;                 
    q_femur = rad2deg(q_femur_rad) + OFFSET_FEMUR + 90 + AJUSTE_FINO_FEMUR_DER; 
    
    % Aplicamos el ajuste fino sumándolo aquí para bajar la tibia
    q_tibia = rad2deg(q_tibia_rad) + OFFSET_TIBIA + 90 + AJUSTE_FINO_TIBIA_DER; 
    
    % --- 7. CORTAFUEGOS DE SEGURIDAD (ANTI-CHOQUE MECÁNICO) ---
    if q_coxa < 5
        q_coxa = 5;
    elseif q_coxa > 175
        q_coxa = 175;
    end
    
    if q_femur < 5
        q_femur = 5;
    elseif q_femur > 175
        q_femur = 175;
    end
    
    if q_tibia < 5
        q_tibia = 5;
    elseif q_tibia > 175
        q_tibia = 175;
    end
end

== matlab function Prueba_Control_Cuadrupedo_Fisico_Imanes/Pata_Derecha_Delantera/MATLAB Function2 ==
  data: cmd input; omega output; Status input
function omega = gait_speed(cmd, Status)
    
    % --- 1. MEMORIA CONTRA EL PARPADEO ---
    persistent cmd_last
    if isempty(cmd_last)
        cmd_last = zeros(3, 1, 'single'); 
    end
    
    if logical(Status) == true
        cmd_last = single(cmd(:)); 
    end
    
    % --- 2. LEER DE LA MEMORIA Y CONVERTIR ---
    % ¡Aquí está el truco! Pasamos al formato 'double' de una vez
    % para que todas las matemáticas fluyan sin errores.
    Vx = double(cmd_last(1));
    Vy = double(cmd_last(2));
    Wz = double(cmd_last(3));
    
    % --- 3. CÁLCULO DE VELOCIDAD ---
    % Ahora 'vel' nace siendo double
    vel = sqrt(Vx^2 + Vy^2 + Wz^2);
    
    % zona muerta
    if vel < 0.1
        vel = 0; % Como 'vel' y '0' son double, ya no hay choque
    end
    
    % frecuencia base del gait
    freq_max = 1.5; 
    omega = vel * freq_max;

== matlab function Prueba_Control_Cuadrupedo_Fisico_Imanes/Pata_Derecha_Delantera/MATLAB Function3 ==
  data: phi input; x_gait output; ID_pata input; y_gait output; z_gait output; vel_x input; vel_y input; iman_estado output
function [x_gait, y_gait, z_gait, iman_estado] = gait_generator(phi, ID_pata, vel_x, vel_y)
% --- 1. POSTURA BASE Y LÍMITES ---
BASE_X = 150;
NOMINAL_Z = -130;
% --- CONFIGURACIÓN DE ALTURA DE PASO UNIFICADA ---
LIFT_Z = -70;
Y_ATRAS = -40;
Y_ADELANTE = 40;
% --- 2. NORMALIZAR EL CICLO Y ORDEN DE MARCHA ---
t_norm = mod(phi, 2*pi) / (2*pi);
switch ID_pata
case 1 % Pata Derecha Delantera
offset = 0.0;
case 2 % Pata Izquierda Trasera
offset = 0.25;
case 3 % Pata Izquierda Delantera
offset = 0.50;
case 4 % Pata Derecha Trasera
offset = 0.75;
otherwise
offset = 0.0;
end
p_local = mod(t_norm - offset, 1.0);
% --- 3. TRAYECTORIA EN 4 FASES (MOVIMIENTO ACTIVO) ---
x_gait = BASE_X;
% FASE 1: DESPEGUE Y VUELO
if p_local < 0.20
s = p_local / 0.20;
s_smooth = 0.5 * (1 - cos(s * pi));
y_gait = Y_ATRAS + (Y_ADELANTE - Y_ATRAS) * s_smooth;
z_gait = NOMINAL_Z + (NOMINAL_Z - LIFT_Z) * -sin(s * pi);
iman_estado_calculado = 0;
% FASE 2: ATERRIZAJE Y ANCLAJE
elseif p_local < 0.25
y_gait = Y_ADELANTE;
z_gait = NOMINAL_Z;
iman_estado_calculado = 1;
% FASE 3: EMPUJE / STANCE
elseif p_local < 0.95
s = (p_local - 0.25) / 0.70;
y_gait = Y_ADELANTE - (Y_ADELANTE - Y_ATRAS) * s;
z_gait = NOMINAL_Z + 10; % Corrección geométrica vertical fija para esta pata
iman_estado_calculado = 1;
% FASE 4: LIBERACIÓN DEL IMÁN
else
y_gait = Y_ATRAS;
z_gait = NOMINAL_Z + 10; % Corrección geométrica vertical fija para esta pata
iman_estado_calculado = 0;
end
% --- 4. CORTAFUEGOS INTELIGENTE: MODO STANDBY TOTAL ---
if abs(vel_x) < 0.1 && abs(vel_y) < 0.1
    x_gait = BASE_X;
    y_gait = 0;
    z_gait = NOMINAL_Z + 10; % Mantiene su altura corregida en reposo
    
    % SOLUCCIÓN DEFINITIVA: Cuando el robot se detiene por completo,
    % obligamos a que el imán se encienda (1) para garantizar que las 4 patas
    % queden totalmente ancladas al suelo en modo estacionario.
    iman_estado = 1; 
    return;
else
    % En movimiento dinámico, sigue la secuencia matemática de las fases
    iman_estado = iman_estado_calculado;
end
end

== matlab function Prueba_Control_Cuadrupedo_Fisico_Imanes/MATLAB Function ==
  data: cmd_raw input size=3; cmd_clean output size=3; Status input boolean
function cmd_clean = Filtro_Maestro(cmd_raw, Status)
    
    % swapbytes voltea los bytes al derecho para arreglar el número e-319
    senial_actual = swapbytes(double(cmd_raw(:)));
    
    % ... (el resto del código se queda igual)
    persistent memoria
    if isempty(memoria)
        memoria = zeros(3, 1, 'double'); 
    end
    
    if logical(Status) == true
        memoria = senial_actual;
    end
    
    cmd_clean = memoria;

== matlab function Prueba_Control_Cuadrupedo_Fisico_Imanes/Pata_Derecha_Trasera/MATLAB Function1 ==
  data: x input; q_coxa output; y input; z input; q_femur output; q_tibia output
function [q_coxa, q_femur, q_tibia] = InverseKinematics(x, y, z)
    % --- 1. CONFIGURACIÓN DEL ROBOT ---
    L1 = 56.84;  % Coxa
    L2 = 80.37;  % Fémur
    L3 = 187.3;  % Tibia 
    
    % --- 2. AJUSTES MANUALES ---
    % Vamos a restar unos 80 grados de golpe para bajar la tibia
    OFFSET_TIBIA = -140;  % (Antes estaba en -40)
    
    % Y por si acaso, bajemos un poco el fémur también
    OFFSET_FEMUR = 30;    % (Antes estaba en 60)
    
    % === CALIBRACIÓN EXCLUSIVA DEL FÉMUR (PATA DERECHA TRASERA) ===
    % MODIFICACIÓN: Sumar grados (+) hace que el fémur baje la pata. 
    % Lo ponemos en 10 para que baje un poquitito nomás.
    % (Si notas que aún le falta bajar un pelo más, súbelo a 15. Si bajó de más, bájalo a 5).
    AJUSTE_FINO_FEMUR_DER = 10;
    
    % --- 3. CÁLCULOS ---
    q_coxa_rad = -atan2(y, x); 
    distancia_xy = sqrt(x^2 + y^2);
    
    R = distancia_xy - L1;
    D = sqrt(R^2 + z^2);
    
    % --- 4. PROTECCIÓN MATEMÁTICA ---
    if D > (L2 + L3)
        D = L2 + L3; 
    end
    D = max(D, abs(L2 - L3) + 1);
    
    cos_alfa = (L2^2 + D^2 - L3^2) / (2 * L2 * D);
    cos_beta = (L2^2 + L3^2 - D^2) / (2 * L2 * L3);
    
    alfa = acos(max(min(cos_alfa, 1), -1));
    beta = acos(max(min(cos_beta, 1), -1));
    elevacion = atan2(z, R); 
    
    % --- 5. CÁLCULO DE ÁNGULOS EN RADIANES ---
    q_femur_rad = -(alfa + elevacion); 
    q_tibia_rad = (pi - beta);         
    
    % --- 6. SALIDA FINAL NORMAL (LADO DERECHO PCA 0x41) ---
    % Aplicamos el ajuste fino únicamente en la línea del fémur
    q_coxa  = rad2deg(q_coxa_rad) + 90;                 
    q_femur = rad2deg(q_femur_rad) + OFFSET_FEMUR + 90 + AJUSTE_FINO_FEMUR_DER; 
    q_tibia = rad2deg(q_tibia_rad) + OFFSET_TIBIA + 90; % Se queda original sin alterar la tibia
    
    % --- 7. CORTAFUEGOS DE SEGURIDAD (ANTI-CHOQUE MECÁNICO) ---
    if q_coxa < 5
        q_coxa = 5;
    elseif q_coxa > 175
        q_coxa = 175;
    end
    
    if q_femur < 5
        q_femur = 5;
    elseif q_femur > 175
        q_femur = 175;
    end
    
    if q_tibia < 5
        q_tibia = 5;
    elseif q_tibia > 175
        q_tibia = 175;
    end
end

== matlab function Prueba_Control_Cuadrupedo_Fisico_Imanes/Pata_Izquierda_Delantera/Locomotion ==
  data: x_gait input; x_final output; y_gait input; z_gait input; Vx input; Vy input; Giro input; ID_pata input; y_final output; z_final output; Status input
function [x_final, y_final, z_final] = fcn(x_gait, y_gait, z_gait, Vx, Vy, Giro, ID_pata, Status)
    
    % --- 1. CONVERSIÓN SEGURA (CORTAFUEGOS) ---
    Vx_d = double(Vx(1));
    Vy_d = double(Vy(1));
    Giro_d = double(Giro(1));
    
    % --- 2. MEMORIA DEL MANDO ---
    persistent Vx_last Vy_last Giro_last
    if isempty(Vx_last)
        Vx_last = 0; Vy_last = 0; Giro_last = 0; 
    end
    
    if logical(Status) == true
        Vx_last = Vx_d;
        Vy_last = Vy_d;
        Giro_last = Giro_d;
    end
    
    % --- 3. FILTRO SUAVIZADOR (ANTI-TEMBLORES) ---
    persistent Vx_f Vy_f Giro_f
    if isempty(Vx_f)
        Vx_f = 0; Vy_f = 0; Giro_f = 0;
    end
    
    % Alpha en 0.15 actúa como amortiguador. Ya no saltará violentamente.
    alpha = 0.15; 
    Vx_f = (1-alpha)*Vx_f + alpha*Vx_last;
    Vy_f = (1-alpha)*Vy_f + alpha*Vy_last;
    Giro_f = (1-alpha)*Giro_f + alpha*Giro_last;
    
    % --- 4. CINEMÁTICA DEL CUERPO Y SALIDA ---
    % Como el gait_generator ya calcula la zancada con vel_x y vel_y,
    % Locomotion solo debe aplicar pequeñas correcciones de postura 
    % o pasar la trayectoria limpia para no deformar el paso.
    
    % Por ahora, pasamos la trayectoria limpia del generador de marcha.
    % Si en el futuro quieres que el cuerpo se incline (body kinematics),
    % se sumaría aquí.
    
    x_final = x_gait;
    y_final = y_gait;
    z_final = z_gait;
end

== matlab function Prueba_Control_Cuadrupedo_Fisico_Imanes/Pata_Izquierda_Delantera/MATLAB Function1 ==
  data: x input; q_coxa output; y input; z input; q_femur output; q_tibia output
function [q_coxa, q_femur, q_tibia] = InverseKinematics(x, y, z)
    % --- 1. CONFIGURACIÓN DEL ROBOT ---
    L1 = 56.84;  % Coxa
    L2 = 80.37;  % Fémur
    L3 = 187.3;  % Tibia 
    
    % --- 2. AJUSTES MANUALES (IGUALADOS A LA TRASERA) ---
    % Sincronizado a -130 grados para que ambas tibias izquierdas partan del mismo punto
    OFFSET_TIBIA = -130;  
    
    % Mantiene la altura base del fémur
    OFFSET_FEMUR = 30;    
    
    % Aplicamos exactamente las mismas calibraciones de la pata trasera
    AJUSTE_FINO_FEMUR_IZQ = -22;
    AJUSTE_FINO_TIBIA_IZQ = -5; 
    
    % --- 3. CÁLCULOS ---
    q_coxa_rad = -atan2(y, x); 
    distancia_xy = sqrt(x^2 + y^2);
    
    R = distancia_xy - L1;
    D = sqrt(R^2 + z^2);
    
    % --- 4. PROTECCIÓN MATEMÁTICA ---
    if D > (L2 + L3)
        D = L2 + L3; 
    end
    D = max(D, abs(L2 - L3) + 1);
    
    cos_alfa = (L2^2 + D^2 - L3^2) / (2 * L2 * D);
    cos_beta = (L2^2 + L3^2 - D^2) / (2 * L2 * L3);
    
    alfa = acos(max(min(cos_alfa, 1), -1));
    beta = acos(max(min(cos_beta, 1), -1));
    elevacion = atan2(z, R); 
    
    % --- 5. CÁLCULO DE ÁNGULOS EN RADIANES ---
    q_femur_rad = -(alfa + elevacion); 
    q_tibia_rad = (pi - beta);         
    
    % --- 6. SALIDA FINAL INVERTIDA (CORREGIDA Y SIMÉTRICA) ---
    % 1ro: Calculamos el ángulo real como si fuera una pata derecha
    femur_derecho = rad2deg(q_femur_rad) + OFFSET_FEMUR + 90;
    tibia_derecha = rad2deg(q_tibia_rad) + OFFSET_TIBIA + 90;
    
    % 2do: Aplicamos el espejo limpio incorporando ambos ajustes finos
    q_coxa  = rad2deg(q_coxa_rad) + 90; 
    q_femur = (180 - femur_derecho) + AJUSTE_FINO_FEMUR_IZQ; % Corregido igual que la trasera
    q_tibia = (180 - tibia_derecha) + AJUSTE_FINO_TIBIA_IZQ;
    
    % --- 7. CORTAFUEGOS DE SEGURIDAD (ANTI-COLAPSO) ---
    if q_tibia < 5
        q_tibia = 5;
    elseif q_tibia > 175
        q_tibia = 175;
    end
    
    if q_femur < 5
        q_femur = 5;
    elseif q_femur > 175
        q_femur = 175;
    end
end

== matlab function Prueba_Control_Cuadrupedo_Fisico_Imanes/Pata_Izquierda_Delantera/MATLAB Function2 ==
  data: cmd input; omega output; Status input
function omega = gait_speed(cmd, Status)
    
    % --- 1. MEMORIA CONTRA EL PARPADEO ---
    persistent cmd_last
    if isempty(cmd_last)
        cmd_last = zeros(3, 1, 'single'); 
    end
    
    if logical(Status) == true
        cmd_last = single(cmd(:)); 
    end
    
    % --- 2. LEER DE LA MEMORIA Y CONVERTIR ---
    % ¡Aquí está el truco! Pasamos al formato 'double' de una vez
    % para que todas las matemáticas fluyan sin errores.
    Vx = double(cmd_last(1));
    Vy = double(cmd_last(2));
    Wz = double(cmd_last(3));
    
    % --- 3. CÁLCULO DE VELOCIDAD ---
    % Ahora 'vel' nace siendo double
    vel = sqrt(Vx^2 + Vy^2 + Wz^2);
    
    % zona muerta
    if vel < 0.1
        vel = 0; % Como 'vel' y '0' son double, ya no hay choque
    end
    
    % frecuencia base del gait
    freq_max = 1.5; 
    omega = vel * freq_max;

== matlab function Prueba_Control_Cuadrupedo_Fisico_Imanes/Pata_Izquierda_Delantera/MATLAB Function3 ==
  data: phi input; x_gait output; ID_pata input; y_gait output; z_gait output; vel_x input; vel_y input; iman_estado output
function [x_gait, y_gait, z_gait, iman_estado] = gait_generator(phi, ID_pata, vel_x, vel_y)
% --- 1. POSTURA BASE Y LÍMITES ---
BASE_X = 150;
NOMINAL_Z = -130;
% --- CONFIGURACIÓN DE ALTURA DE PASO UNIFICADA ---
LIFT_Z = -70;
Y_ATRAS = -40;
Y_ADELANTE = 40;
% --- 2. NORMALIZAR EL CICLO Y ORDEN DE MARCHA ---
t_norm = mod(phi, 2*pi) / (2*pi);
switch ID_pata
case 1 % Pata Derecha Delantera
offset = 0.0;
case 2 % Pata Izquierda Trasera
offset = 0.25;
case 3 % Pata Izquierda Delantera
offset = 0.50;
case 4 % Pata Derecha Trasera
offset = 0.75;
otherwise
offset = 0.0;
end
p_local = mod(t_norm - offset, 1.0);
% --- 3. TRAYECTORIA EN 4 FASES (MOVIMIENTO ACTIVO) ---
x_gait = BASE_X;
% FASE 1: DESPEGUE Y VUELO
if p_local < 0.20
s = p_local / 0.20;
s_smooth = 0.5 * (1 - cos(s * pi));
y_gait = Y_ATRAS + (Y_ADELANTE - Y_ATRAS) * s_smooth;
z_gait = NOMINAL_Z + (NOMINAL_Z - LIFT_Z) * -sin(s * pi);
iman_estado_calculado = 0;
% FASE 2: ATERRIZAJE Y ANCLAJE
elseif p_local < 0.25
y_gait = Y_ADELANTE;
z_gait = NOMINAL_Z;
iman_estado_calculado = 1;
% FASE 3: EMPUJE / STANCE
elseif p_local < 0.95
s = (p_local - 0.25) / 0.70;
y_gait = Y_ADELANTE - (Y_ADELANTE - Y_ATRAS) * s;
z_gait = NOMINAL_Z + 10; % Corrección geométrica vertical fija para esta pata
iman_estado_calculado = 1;
% FASE 4: LIBERACIÓN DEL IMÁN
else
y_gait = Y_ATRAS;
z_gait = NOMINAL_Z + 10; % Corrección geométrica vertical fija para esta pata
iman_estado_calculado = 0;
end
% --- 4. CORTAFUEGOS INTELIGENTE: MODO STANDBY TOTAL ---
if abs(vel_x) < 0.1 && abs(vel_y) < 0.1
    x_gait = BASE_X;
    y_gait = 0;
    z_gait = NOMINAL_Z + 10; % Mantiene su altura corregida en reposo
    
    % SOLUCCIÓN DEFINITIVA: Cuando el robot se detiene por completo,
    % obligamos a que el imán se encienda (1) para garantizar que las 4 patas
    % queden totalmente ancladas al suelo en modo estacionario.
    iman_estado = 1; 
    return;
else
    % En movimiento dinámico, sigue la secuencia matemática de las fases
    iman_estado = iman_estado_calculado;
end
end

== matlab function Prueba_Control_Cuadrupedo_Fisico_Imanes/Pata_Izquierda_Trasera/Locomotion ==
  data: x_gait input; x_final output; y_gait input; z_gait input; Vx input; Vy input; Giro input; ID_pata input; y_final output; z_final output; Status input
function [x_final, y_final, z_final] = fcn(x_gait, y_gait, z_gait, Vx, Vy, Giro, ID_pata, Status)
    
    % --- 1. CONVERSIÓN SEGURA (CORTAFUEGOS) ---
    Vx_d = double(Vx(1));
    Vy_d = double(Vy(1));
    Giro_d = double(Giro(1));
    
    % --- 2. MEMORIA DEL MANDO ---
    persistent Vx_last Vy_last Giro_last
    if isempty(Vx_last)
        Vx_last = 0; Vy_last = 0; Giro_last = 0; 
    end
    
    if logical(Status) == true
        Vx_last = Vx_d;
        Vy_last = Vy_d;
        Giro_last = Giro_d;
    end
    
    % --- 3. FILTRO SUAVIZADOR (ANTI-TEMBLORES) ---
    persistent Vx_f Vy_f Giro_f
    if isempty(Vx_f)
        Vx_f = 0; Vy_f = 0; Giro_f = 0;
    end
    
    % Alpha en 0.15 actúa como amortiguador. Ya no saltará violentamente.
    alpha = 0.15; 
    Vx_f = (1-alpha)*Vx_f + alpha*Vx_last;
    Vy_f = (1-alpha)*Vy_f + alpha*Vy_last;
    Giro_f = (1-alpha)*Giro_f + alpha*Giro_last;
    
    % --- 4. CINEMÁTICA DEL CUERPO Y SALIDA ---
    % Como el gait_generator ya calcula la zancada con vel_x y vel_y,
    % Locomotion solo debe aplicar pequeñas correcciones de postura 
    % o pasar la trayectoria limpia para no deformar el paso.
    
    % Por ahora, pasamos la trayectoria limpia del generador de marcha.
    % Si en el futuro quieres que el cuerpo se incline (body kinematics),
    % se sumaría aquí.
    
    x_final = x_gait;
    y_final = y_gait;
    z_final = z_gait;
end
